simulink model "ardupilotsailboat"  (R2022b)
settings: Solver=VariableStepAuto  StartTime=0.0  StopTime=85  RelTol=1e-3
values from neighbouring files (symbols this model uses):
  m11 = 0.1    [ThreeDOF.m]
  m22 = 0.1    [ThreeDOF.m]
undefined symbols (not defined in the file or in its folder): Ixx, m, Waypoints, Yv
libraries: cstblocks x2, simulink x1
(part 2 of 2)

== matlab function ardupilotsailboat/Subsystem8/MATLAB Function ==
  data: u input; y output; max input
function y = fcn(u,max)
if u>max
    u=max;
else 
    if u<-max
        u=-max;
    end
end
y = u;

== matlab function ardupilotsailboat/Subsystem7/MATLAB Function ==
  data: u input; y output; max input; min input
function y = fcn(u,max,min)
if u>max
    u=max;
else 
    if u<min
        u=min;
    end
end
y = u;

== matlab function ardupilotsailboat/Subsystem3/MATLAB Function14 ==
  data: beta input; wu output; wv output; wr output; t input
function [wu,wv,wr] = WaveForcesandMoments(beta,t)
% Water density (kg/m^2)
rho = 1025;

% Gravity (m/s^2)
g = 9.81;

% Vessel size (m)
L = 2;
B = 0.125;
T = 0.4;

% Vessels Heading

% Wave Specifications
% amplitude(m)
Ai = 0.4;
% length(m)
lamdai = 5;
% encounter frequency (rads)
omegai = 0.4;
% random phase (rads)
phii = -pi;

% Wave Component
waveC = Ai * (2*pi)/lamdai * sin(omegai*t + phii);

% u Component
wu = (10^(-6)) * rho * g * B * L * T * cos(beta) * waveC;

% v Component
wv = (10^(-6)) * rho * g * B * L * T * sin(beta) * waveC;

% r Component
wr = (10^(-6)) * 1/24 * rho * g * B * L * (L^2 - B^2) * sin(2*beta) * waveC^2;

== matlab function ardupilotsailboat/Subsystem3/MATLAB Function15 ==
  data: windDirect input; wi_u output; wi_v output; wi_r output; V_w input; psi input; u input; v input
function [wi_u,wi_v,wi_r] = WindForcesandMoments(windDirect,V_w,psi,u,v)
% Air density (kg/m^2)
rho = 1.225;

% Ship Size
L = 2;
B = 0.125;
T = 0.4;

% centroids above the water line of the frontal and lateral projected areas
H_fw = T - 1.2;
H_lw = T - 1.2;
A_fw = B * H_fw;
A_lw = L * H_lw;


% Symmetrical Ship Coeff
c_x = 0.7;
c_y = 0.825;
c_r = 0.125;

% Wind Velocities in x- and y-coordinates
u_w = V_w * cos(windDirect - psi);
v_w = V_w * sin(windDirect - psi);

% Relative wind velocities
u_rw = u - u_w;
v_rw = v - v_w;

% Relative Wind Velocity and direction
V_rw = sqrt(u_rw^2 + v_rw^2);
gamma_rw = -atan(v_rw/u_rw);

% Wind Coeff
C_x = -c_x * cos(gamma_rw);
C_y = c_y * sin(gamma_rw);
C_r = c_r * sin(2*gamma_rw);

% Wind Forces and Moments
wi_u = 0.5 * rho * V_rw *  C_x * A_fw * 10^(-2);
wi_v = 0.5 * rho * V_rw *  C_y * A_lw * 10^(-2);
wi_r = 0.5 * rho * V_rw *  C_r * A_lw * 10^(-2);

== matlab function ardupilotsailboat/MATLAB Function3 ==
  data: delta_s input; apparent_velocity input; Xs output; Ys output; Ks output; Ns output; awa output; apparent_wind_angle input; phi input
function [Xs,Ys,Ks,Ns,awa] = sailForce(delta_s,apparent_velocity,apparent_wind_angle,phi)
%Parameters
rho_a = 1.2;
area_sail =0.38;
l1 =0;
l2 = 0;
h1 = 0.6;

% CoE of sail
zs = 0.6;
xs=0;
ys=0;

% Apparent Wind Velocity
awa=apparent_wind_angle;

% Calculate Angle of Attack
alpha = awa-delta_s;


% Calculate Lift and Drag Force
[Cls,Cds] = sailcoef(alpha);
Ls = 0.5*rho_a*area_sail*(apparent_velocity)*Cls;
Ds = 0.5*rho_a*area_sail*(apparent_velocity)*Cds;

% Sail Force components
Xs = (Ls * sin(awa) - Ds * cos(awa));
Ys = (Ls * cos(awa) + Ds * sin(awa));
Ks =- h1 *(Ls * cos(awa) + Ds * sin(awa));
Ns = (-Xs * l2 * sin(delta_s) + Ys*(l1 - l2*cos(delta_s)));

function [Cls,Cds] = sailcoef(attack)
% generate a lookup table for the lift/drag coefficients for the sail
% and compute Cls/Cds from the lookup table using interpolation.

% lookup table
xdata = linspace(-pi,pi,73); % every 5 degrees
xdata = xdata/pi*180;

% lift curve
yldata = [fliplr([0 0.15 0.32 ...
    0.48 0.7 0.94 1.15 1.3 1.28 1.15 1.1 1.05 1 0.9 0.82 0.72 0.68 0.56 0.48 0.32 0.21 0.08 ...
    -0.06 -0.18 -0.3 -0.4 -0.53 -0.64 -0.72 -0.84 -0.95 -1.04 -1.1 -1.14 -1.08 -0.76 0])*(-1) ...
    [0.15 0.32 ...
    0.48 0.7 0.94 1.15 1.3 1.28 1.15 1.1 1.05 1 0.9 0.82 0.72 0.68 0.56 0.48 0.32 0.21 0.08 ...
    -0.06 -0.18 -0.3 -0.4 -0.53 -0.64 -0.72 -0.84 -0.95 -1.04 -1.1 -1.14 -1.08 -0.76 0]];

% drag curve
yddata = [fliplr([0.1 0.12 0.14 ...
    0.16 0.19 0.26 0.35 0.46 0.54 0.62 0.7 0.78 0.9 0.98 1.04 1.08 1.16 1.2 1.24 1.26 ...
    1.28 1.34 1.36 1.37 1.33 1.31 1.28 1.26 1.25 1.2 1.1 1.04 0.88 0.8 0.64 0.38 0.1])...
    [0.12 0.14 ...
    0.16 0.19 0.26 0.35 0.46 0.54 0.62 0.7 0.78 0.9 0.98 1.04 1.08 1.16 1.2 1.24 1.26 ...
    1.28 1.34 1.36 1.37 1.33 1.31 1.28 1.26 1.25 1.2 1.1 1.04 0.88 0.8 0.64 0.38 0.1]];

% fit the input angle of attack into the interval [-pi,pi]
if attack > pi
    attack = mod(attack+pi,2*pi) - pi;
else
    if attack < -pi
        attack = mod(attack-pi,-2*pi) + pi;
    end
end

% interpolation
attack = attack/pi*180;
Cls = interp1(xdata,yldata,attack,'pchip');
Cds = interp1(xdata,yddata,attack,'pchip');
